simulink model "HW_1_VM"  (R2020a)
settings: Solver=ode3  StartTime=0.0  StopTime=simPrm.tEnd  FixedStep=simPrm.dt  MaxStep=1/30  RelTol=1e-3  EnableMultiTasking=on
values from neighbouring files (symbols this model uses):
  A = [calc.Z1 calc.Z2     0     0   0 ... (first row only)    [HW1_VMsetup.m]
  B = [1/Motor.La; 0; 0; 0; 0]    [HW1_VMsetup.m]
  C = [0 0 0 0 1 ... (first row only)    [HW1_VMsetup.m]
  D = [0;0;0;0;0;0]    [HW1_VMsetup.m]
  g = 9.81    [HW1_VMsetup.m]
undefined symbols (not defined in the file or in its folder): calc, Gear, Load, Motor
libraries: simulink_extras x2
settings Model: Creator=ggparker  LastModifiedBy=vmali
settings DataIOCC: LimitDataPoints=on
settings OptimizationCC: LifeSpan=inf
settings DebuggingCC: AllowSymbolicDim=off  SFUnexpectedBacktrackingDiag=warning  SFNoUnconditionalDefaultTransitionDiag=warning  SFExecutionAtInitializationDiag=none  ArithmeticOperatorsInVariantConditions=warning
settings SFSimCC: SimUseLocalCustomCode=off  CustomCodeUndefinedFunction=UseInterfaceOnly
settings RTWCC: RTWUseLocalCustomCode=off
settings CodeAppCC: StateflowObjectComments=on
settings GRTTargetCC: TargetLangStandard=C89/C90 (ANSI)
settings ConfigComp: CovMetricSettings=dw  CovHtmlReporting=on  CovSaveCumulativeToWorkspaceVar=on  CovSaveSingleToWorkspaceVar=on  CovExternalEMLEnable=off  CovSFcnEnable=off
settings SimscapeCC: SimscapeNominalValues="[{\"value\":\"10\",\"unit\":\"V\"},{\"value\":\"1\",\"unit\":\"A\"},{\"value\":\"10\",\"unit\":\"N*m\"},{\"value\":\"10\",\"unit\":\"bar\"},{\"value\":\"100\",\"unit\":\"kJ/kg\"},{\"value\":\"1\",\"unit\":\"kW\"},{\"value\":\"300\",\"unit\":\"K\"},{\"value\":\"100\",\"unit\":\"cm^3/s\"},{\"value\":\"1\",\"unit\":\"kN\"},{\"value\":\"1\",\"unit\":\"g/cm^3\"},{\"value\":\"1\",\"unit\":\"l\"},{\"value\":\"1\",\"unit\":\"cm^2\"},{\"value\":\"60\",\"unit\":\"Hz\"}]"  SimscapeLogType=all  SimscapeLogToSDI=on  SimscapeLogDataHistory=10000
settings ConfigurationSet: Description=SimMechanics 2G

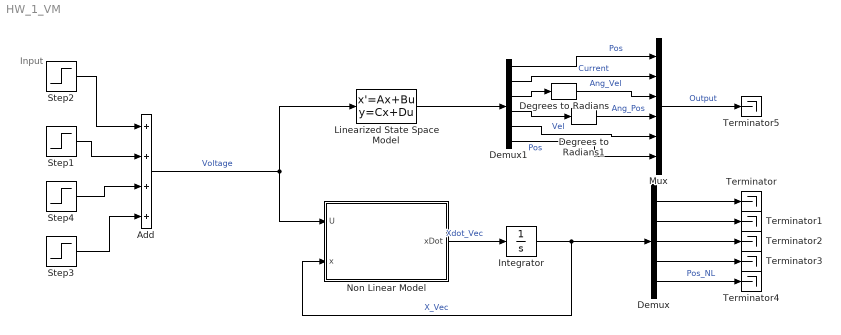
== system HW_1_VM ==
  note: Input
  Add : Sum  Inputs=++++
  Degrees to Radians : simulink_extras/Transformations/Degrees to Radians
  Degrees to Radians1 : simulink_extras/Transformations/Degrees to Radians
  Demux : Demux  Outputs=5
  Demux1 : Demux  Outputs=6
  Integrator : Integrator  InitialCondition=[0;0;0;0;0]
  Linearized State Space Model : StateSpace  A=A  B=B  C=C  D=D  InitialCondition=[0;0;0;0;0]  ContinuousStateAttributes={'Current', 'Ang_Accl', 'Ang_Vel','Acc','Vel'}
  Mux : Mux  Inputs=6
  Non Linear Model : MATLAB Function  TreatAsAtomicUnit=on
  Step1 : Step  Time=5  After=-200  SampleTime=0
      settings: AttributesFormatString=%<After>
  Step2 : Step  Time=0  After=200  SampleTime=0
      settings: AttributesFormatString=Amp = %<After>
  Step3 : Step  Time=15  After=-200  SampleTime=0
      settings: AttributesFormatString=%<After>
  Step4 : Step  Time=10  After=200  SampleTime=0
      settings: AttributesFormatString=Amp = %<After>
  Terminator{,1..5} (6 alike) : Terminator
  wires:
  Step2/1 -> Add/1
  Step1/1 -> Add/2
  Step4/1 -> Add/3
  Step3/1 -> Add/4
  Non Linear Model/1(xDot) -> Integrator/1  "Xdot_Vec"
  Integrator/1 -> Non Linear Model/2(x), Demux/1  "X_Vec"
  Demux/1 -> Terminator/1
  Demux/2 -> Terminator1/1
  Demux/3 -> Terminator2/1
  Demux/4 -> Terminator3/1
  Demux/5 -> Terminator4/1  "Pos_NL"
  Add/1 -> Non Linear Model/1(U), Linearized State Space Model/1  "Voltage"
  Linearized State Space Model/1 -> Demux1/1
  Demux1/1 -> Mux/1  "Pos"
  Demux1/2 -> Mux/2  "Current"
  Demux1/3 -> Degrees to Radians/1
  Demux1/4 -> Degrees to Radians1/1
  Demux1/5 -> Mux/5  "Vel"
  Demux1/6 -> Mux/6  "Pos"
  Mux/1 -> Terminator5/1  "Output"
  Degrees to Radians/1 -> Mux/3  "Ang_Vel"
  Degrees to Radians1/1 -> Mux/4  "Ang_Pos"

== matlab function HW_1_VM/Non Linear Model ==
  data: U input; x input size=5; xDot output size=5; Motor parameter; calc parameter; Load parameter; g parameter; Gear parameter
function xDot = f(U,x,Motor,calc,Load,g, Gear)
% Function f of x' = f(x)
% x == states

% grab memory
xDot = zeros(5,1);

% Create the xDot equations

xDot(1) = U/Motor.La -(Motor.Ra/Motor.La)*x(1) -(Motor.Ke/Motor.La)*x(2) ;  % Armature current
xDot(2) = (Motor.Ka*x(1)*calc.N^2 - x(3)*Load.K*Gear.Rw^2 + Load.K*calc.N*Gear.Rw*x(5))/Motor.Jm;  % Angular acceleration of motor shaft
xDot(3) = x(2);  % Angular Velocity of motor shaft
xDot(4) = -g + (Load.K*Gear.Rw*x(3))/(Load.M*calc.N) - (Load.K*x(5)/Load.M);  % Accelaration of elevator car
xDot(5) = x(4);  % Velocity of motor car
